simulink model "CANsimple"  (R2017b)
settings: Solver=VariableStepAuto  StartTime=0.0  StopTime=10.0  RelTol=1e-3
libraries: truetime x3
settings Model: Creator=ECC  LastModifiedBy=ECC

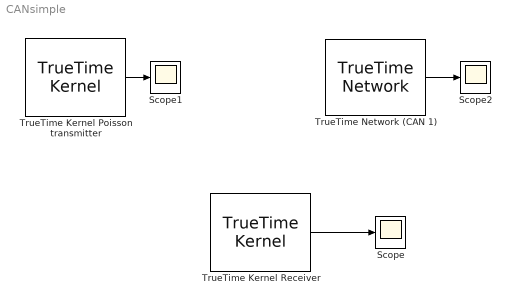
== system CANsimple ==
  Scope : Scope
  Scope1 : Scope
  Scope2 : Scope
  TrueTime Kernel Poisson transmitter : truetime/TrueTime Kernel  Priority=1  sfun=disturbance_init1  args=[]  ninputsoutputs=[0 0]  ntriggers=0  trigtype=rising  nwnodenbr=[1 1]  clockoffsetdrift=[0 0]  schedoutput=on  battery=off  poweroutput=off  label=1: 1
  TrueTime Kernel Receiver : truetime/TrueTime Kernel  Priority=1  sfun=receiver_init  args=[]  ninputsoutputs=[0 1]  ntriggers=0  trigtype=rising  nwnodenbr=[1 2]  clockoffsetdrift=[0 0]  schedoutput=off  battery=off  poweroutput=off  label=1: 2
  TrueTime Network (CAN 1) : truetime/TrueTime Network  Priority=1  nwtype=CSMA/AMP (CAN)  nwnbr=1  nnodes=2  rate=125000  minsize=29  lossprob=0  seed=0  bandwidths=[0.5 0.25 0.25]  slotsize=80  schedule=[1 2 1 3]  memsize=80000  buftype=Common buffer  overflow=Retransmit  dynSchedule=[]  miniSlotSize=40  NIT=0  QSortMode=FIFO  sync=0  irtSchedule=0  nrtLength=0  nodeGraph=0  scheduleoutput=on
  wires:
  TrueTime Network (CAN 1)/1 -> Scope2/1
  TrueTime Kernel Receiver/1 -> Scope/1
  TrueTime Kernel Poisson transmitter/1 -> Scope1/1
